simulink model "LAB4"  (R2023b)
settings: Solver=FixedStepDiscrete  StartTime=0.0  StopTime=Inf  FixedStep=0.02  RelTol=1e-3  EnableMultiTasking=on
model workspace (MAT data in the model file):
  SL_ROS_VariableLengthArrays_MaxSizes.CommonInfo.ArrayTruncateAction = 'EmitWarning'
  SL_ROS_VariableLengthArrays_MaxSizes.MsgTypeMap = containers.Map
  SL_ROS_VariableLengthArrays_MaxSizes.MsgTypeMap.serialization.keys = {'sensor_msgs/LaserScan'}
  SL_ROS_VariableLengthArrays_MaxSizes.MsgTypeMap.serialization.values{1}(1).PropertyName = 'Intensities'
  SL_ROS_VariableLengthArrays_MaxSizes.MsgTypeMap.serialization.values{1}(1).DataType = 'single'
  SL_ROS_VariableLengthArrays_MaxSizes.MsgTypeMap.serialization.values{1}(1).MaxLength = 360
  SL_ROS_VariableLengthArrays_MaxSizes.MsgTypeMap.serialization.values{1}(2).PropertyName = 'Ranges'
  SL_ROS_VariableLengthArrays_MaxSizes.MsgTypeMap.serialization.values{1}(2).DataType = 'single'
  SL_ROS_VariableLengthArrays_MaxSizes.MsgTypeMap.serialization.values{1}(2).MaxLength = 360
  SL_ROS_VariableLengthArrays_MaxSizes.MsgTypeMap.serialization.uniformity = 0
  SL_ROS_VariableLengthArrays_MaxSizes.MsgTypeMap.serialization.keyType = 'char'
  SL_ROS_VariableLengthArrays_MaxSizes.MsgTypeMap.serialization.valueType = 'any'
values from neighbouring files (symbols this model uses):
  x = x + offset    [lab4.m]    (also in occupancy_map.m; occupancy_map2.m)
  x_path = x_path(4:4:end)    [lab4.m]
  y = y + offset    [lab4.m]    (also in occupancy_map.m; occupancy_map2.m)
  y_path = y_path(4:4:end)    [lab4.m]
undefined symbols (not defined in the file or in its folder): angdiff, Angular, Linear
libraries: simulink x5, robotlib x4, robotcorelib x1, simulink_extras x1
(part 1 of 2)
settings Model: Creator=The MathWorks, Inc.  LastModifiedBy=hampu
settings SolverCC: AlgebraicLoopSolver=TrustRegion
settings DataIOCC: LimitDataPoints=on  SaveFormat=Array  ReturnWorkspaceOutputs=off
settings OptimizationCC: ZeroExternalMemoryAtStartup=off  ZeroInternalMemoryAtStartup=off  LifeSpan=Inf  MaxStackSize=64
settings DebuggingCC: SolverPrmCheckMsg=warning  UnconnectedInputMsg=warning  UnconnectedOutputMsg=warning  UnconnectedLineMsg=warning  AllowSymbolicDim=off  SFUnexpectedBacktrackingDiag=warning  SFNoUnconditionalDefaultTransitionDiag=warning  SFExecutionAtInitializationDiag=none  ArithmeticOperatorsInVariantConditions=warning
settings HardwareCC: ProdBitPerPointer=32  ProdBitPerSizeT=32  ProdBitPerPtrDiffT=32  ProdLargestAtomicFloat=None  ProdIntDivRoundTo=Undefined  ProdEndianess=Unspecified  ProdWordSize=32  ProdHWDeviceType=Generic->Unspecified (assume 32-bit Generic)  TargetHWDeviceType=Generic->Unspecified (assume 32-bit Generic)  UseEmbeddedCoderFeatures=off
settings ModelReferenceCC: EnableRefExpFcnMdlSchedulingChecks=on  PropagateSignalLabelsOutOfModel=off
settings SFSimCC: SimUseLocalCustomCode=off  CustomCodeUndefinedFunction=UseInterfaceOnly  SimTargetLang=C++
settings RTWCC: Description=Embedded Coder  SystemTargetFile=ert.tlc  HardwareBoard=Robot Operating System (ROS)  TemplateMakefile=ert_default_tmf  RTWUseLocalCustomCode=off  Toolchain=Catkin  TargetLang=C++
settings CodeAppCC: StateflowObjectComments=on
settings ERTTargetCC: MultiwordLength=2048  ERTCustomFileBanners=off  CodeInterfacePackaging=C++ class  SupportContinuousTime=on  SupportNonInlinedSFcns=on  RemoveResetFunc=off  SupportVariableSizeSignals=on  ModelStepFunctionPrototypeControlCompliant=off  RootIOFormat=Structure reference  ConvertIfToSwitch=off  SuppressUnreachableDefaultCases=off
settings ConfigComp: CovMetricSettings=dw  CovSaveCumulativeToWorkspaceVar=on  CovSaveSingleToWorkspaceVar=on  CovExternalEMLEnable=off  CovSFcnEnable=off

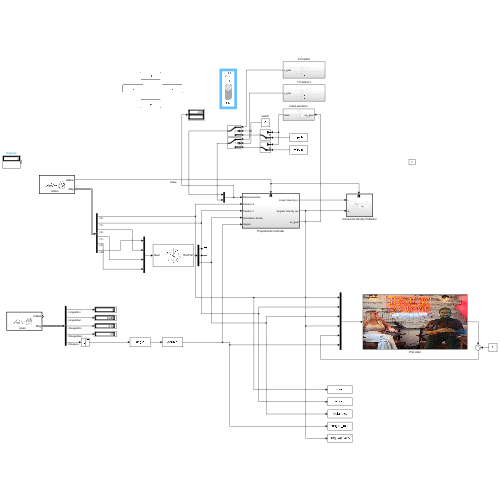
[thumbnail: Simulink's stored preview of the top-level diagram]
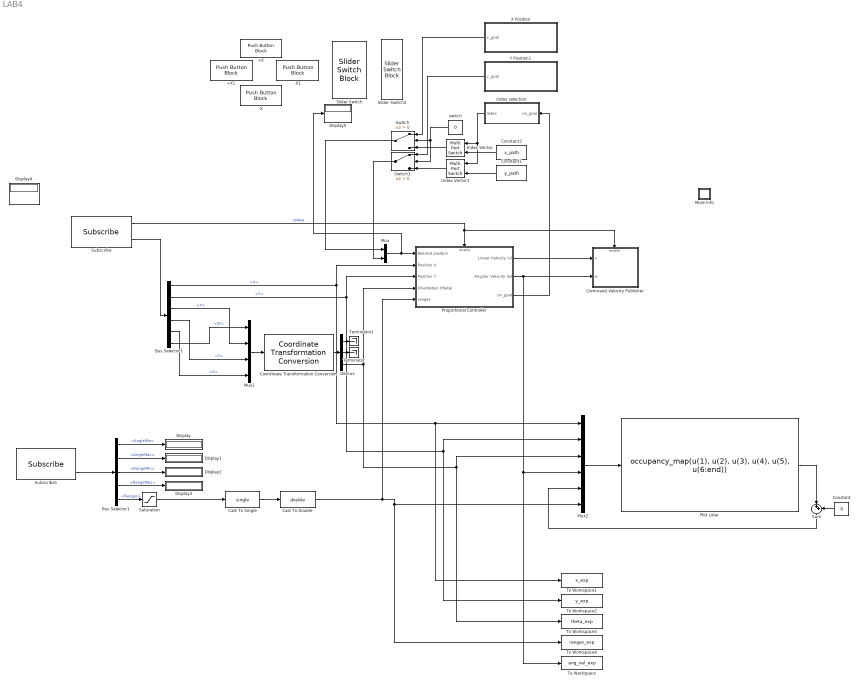
== system LAB4 ==
  +X : PushButtonBlock  ButtonText=+x  CustomIcon=data:image/png;base64,iVBORw0KGgoAAAANSUhEUgAAAdEAAAJTCAYAAABXUyzVAAAAAXNSR0IArs4c6QAAAARnQU1BAACxjwv8YQUAAAAJcEhZcwAAEnQAABJ0Ad5mH3gAAP+lSURBVHhehP13ux21sr4L81ne6z3nt1cADE5zeuacs3POERMM2IAx2eScMyYvcgYHsMERR3AgrL3Pd6nz3NJ45pAH3uv8UZekUqmk7jGn7i51t/qyY8f3x9Gff5iUw0f3xc8nDgR6hPzxkz9O5ku965Ay7/Kx4wfi5OmDcezUT3Hs9E9x9JT8KP35zME4fEL9qnz0ZG6HnX2ckL39nJAeuyOyo63bH//lUM5LjlOW3clfDiuVjex/lo+TssHvSezk+9SZQ5P+T2BT0Vnv/mmTbbJkH1lH ...(+721780 chars)  OffValue=0.000000
  +X1 : PushButtonBlock  ButtonText=+y  OffValue=0.000000
  -X : PushButtonBlock  ButtonText=-x  OffValue=0.000000
  -X1 : PushButtonBlock  ButtonText=-y  OffValue=0.000000
  Bus Selector1 : BusSelector  OutputSignals=AngleMin,AngleMax,RangeMin,RangeMax,Ranges
  Bus Selector3 : BusSelector  OutputSignals=Pose.Pose.Position.X,Pose.Pose.Position.Y,Pose.Pose.Orientation.X,Pose.Pose.Orientation.Y,Pose.Pose.Orientation.Z,Pose.Pose.Orientation.W
  Cast To Double : DataTypeConversion  OutDataTypeStr=double  SaturateOnIntegerOverflow=off  RndMeth=Floor
  Cast To Single : DataTypeConversion  OutDataTypeStr=single  SaturateOnIntegerOverflow=off  RndMeth=Floor
  Command Velocity Publisher : Subsystem
  Constant : Constant  Value=0
  Constant1 : Constant  Value=y_path
  Constant2 : Constant  Value=x_path
  Coordinate Transformation Conversion : robotcorelib/Coordinate Transformation Conversion  InputRepresentation=Quaternion  InputEulerSequence=ZYX  ShowTrVecInputPort=on  OutputRepresentation=Euler Angles  OutputEulerSequence=XYZ  ShowTrVecOutputPort=on  SimulateUsing=Interpreted execution
      settings: LibrarySourceBlock=roslib/Utilities/Coordinate Transformation Conversion
  Demux : Demux  Outputs=3
  Display{,1..5} (6 alike) : Display
  Index Vector : MultiPortSwitch  DataPortOrder=Zero-based contiguous  Inputs=1  zeroidx=on  SaturateOnIntegerOverflow=off  InputSameDT=off
  Index Vector1 : MultiPortSwitch  DataPortOrder=Zero-based contiguous  Inputs=1  zeroidx=on  SaturateOnIntegerOverflow=off  InputSameDT=off
  More Info : Subsystem
      settings: OpenFcn=showdemo(bdroot(gcb))
      mask Display: disp('?')
  Mux : Mux  Inputs=2
  Mux1 : Mux
  Mux2 : Mux  Inputs=6
  Plot Lidar : MATLABFcn  MATLABFcn=occupancy_map(u(1), u(2), u(3), u(4), u(5), u(6:end))
      mask Display: image('bardia_tuah.png');
  Proportional Controller : Subsystem
  Saturation : Saturate  UpperLimit=3.5  LowerLimit=0.12  LinearizeAsGain=off
  Slider Switch : SliderSwitchBlock
      settings: Values={{'TRAJ', 'MANUAL'}, [0 1]}
  Slider Switch2 : SliderSwitchBlock
      settings: Values={{'ON', 'OFF'}, [0 1]}
  Subscribe : robotlib/Subscribe  topicSource=Select from ROS network  topic=/odom  messageType=nav_msgs/Odometry  SampleTime=-1  legacyBusStruct=off  messageQueueLength=51
  Subscribe1 : robotlib/Subscribe  topicSource=Select from ROS network  topic=/scan  messageType=sensor_msgs/LaserScan  SampleTime=-1  legacyBusStruct=off  messageQueueLength=51
  Sum : Sum  Inputs=|++
  Switch : Switch  Criteria=u2 > Threshold  SaturateOnIntegerOverflow=off  InputSameDT=off
  Switch1 : Switch  Criteria=u2 > Threshold  SaturateOnIntegerOverflow=off  InputSameDT=off
  Terminator : Terminator
  Terminator1 : Terminator
  To Workspace : ToWorkspace  VariableName=ang_vel_exp  SaveFormat=Timeseries  SampleTime=-1
  To Workspace1 : ToWorkspace  VariableName=x_exp  SaveFormat=Timeseries  SampleTime=-1
  To Workspace2 : ToWorkspace  VariableName=y_exp  SaveFormat=Timeseries  SampleTime=-1
  To Workspace3 : ToWorkspace  VariableName=theta_exp  SaveFormat=Timeseries  SampleTime=-1
  To Workspace4 : ToWorkspace  VariableName=ranges_exp  SaveFormat=Timeseries  SampleTime=-1
  X Position : Subsystem
  Y Position1 : Subsystem
  index selection : Subsystem
  switch : Constant  Value=0
  wires:
  Subscribe/2 -> Bus Selector3/1
  Proportional Controller/1(Linear Velocity (v)) -> Command Velocity Publisher/1(v)
  Subscribe/1 -> Command Velocity Publisher/Enable, Proportional Controller/Enable  "IsNew"
  Bus Selector3/3 -> Mux1/2  "<X>"
  Bus Selector3/4 -> Mux1/3  "<Y>"
  Bus Selector3/5 -> Mux1/4  "<Z>"
  Bus Selector3/6 -> Mux1/1  "<W>"
  Bus Selector3/2 -> To Workspace2/1, Mux2/2, Proportional Controller/3(Position Y)  "<Y>"
  Bus Selector3/1 -> Proportional Controller/2(Position X), To Workspace1/1, Mux2/1  "<X>"
  X Position/1(x_goal) -> Switch/1
  Y Position1/1(y_goal) -> Switch1/1
  Mux/1 -> Proportional Controller/1(Desired position), Display5/1
  Mux1/1 -> Coordinate Transformation Conversion/1
  Coordinate Transformation Conversion/1 -> Demux/1
  Demux/3 -> To Workspace3/1, Mux2/3, Proportional Controller/4(Orientation (theta))
  Demux/1 -> Terminator1/1
  Demux/2 -> Terminator/1
  Bus Selector1/2 -> Display1/1  "<AngleMax>"
  Bus Selector1/4 -> Display3/1  "<RangeMax>"
  Bus Selector1/1 -> Display/1  "<AngleMin>"
  Bus Selector1/3 -> Display2/1  "<RangeMin>"
  Subscribe1/2 -> Bus Selector1/1
  Bus Selector1/5 -> Saturation/1  "<Ranges>"
  Saturation/1 -> Cast To Single/1
  Cast To Single/1 -> Cast To Double/1
  Cast To Double/1 -> Proportional Controller/5(ranges), To Workspace4/1, Mux2/6
  Mux2/1 -> Plot Lidar/1
  Proportional Controller/2(Angular Velocity (w)) -> To Workspace/1, Mux2/4, Command Velocity Publisher/2(w)
  Plot Lidar/1 -> Sum/1
  Constant/1 -> Sum/2
  Sum/1 -> Mux2/5
  Proportional Controller/3(on_goal) -> index selection/1(on_goal)
  Constant2/1 -> Index Vector/2
  Constant1/1 -> Index Vector1/2
  index selection/1(index) -> Index Vector1/1, Index Vector/1
  Index Vector1/1 -> Switch1/3
  Index Vector/1 -> Switch/3
  Switch/1 -> Mux/1
  Switch1/1 -> Mux/2
  switch/1 -> Switch/2, Switch1/2
